simulink model "Linearni"  (R2023b)
settings: Solver=VariableStepAuto  StartTime=0.0  StopTime=stepp.sim_time  RelTol=1e-3
undefined symbols (not defined in the file): ccm_op, dcm_op_cv, G_ccm, Gp_dcm_cv, stepp
settings Model: Creator=teo  LastModifiedBy=teo

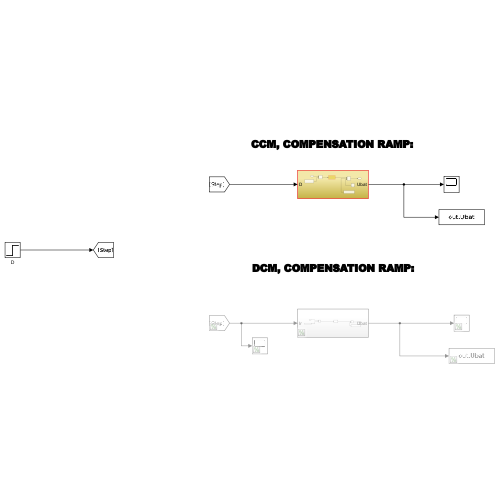
[thumbnail: Simulink's stored preview of the top-level diagram]
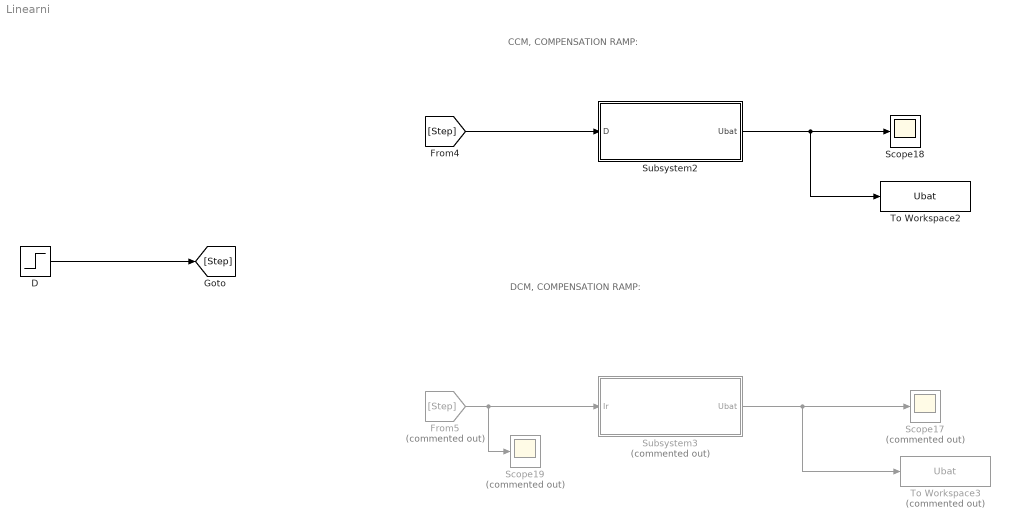
== system Linearni ==
  note: CCM, COMPENSATION RAMP:
  note: DCM, COMPENSATION RAMP:
  D : Step  Time=stepp.step_time  Before=stepp.D1  After=stepp.D2  SampleTime=0
  From5 : From  Commented=on  GotoTag=Step
  Scope17 : Scope  Commented=on
  Scope18 : Scope
  Scope19 : Scope  Commented=on
  Subsystem2 : Subsystem
  Subsystem3 : Subsystem  Commented=on
  To Workspace2 : ToWorkspace  VariableName=Ubat  SaveFormat=Timeseries  SampleTime=1e-6
  To Workspace3 : ToWorkspace  Commented=on  VariableName=Ubat  SaveFormat=Timeseries  SampleTime=1e-6
  wires:
  [Step] -> Subsystem2/1(D)
  Subsystem2/1(Ubat) -> Scope18/1, To Workspace2/1
  From5/1 -> Scope19/1, Subsystem3/1(Ir)
  Subsystem3/1(Ubat) -> To Workspace3/1, Scope17/1
  D/1 -> [Step]

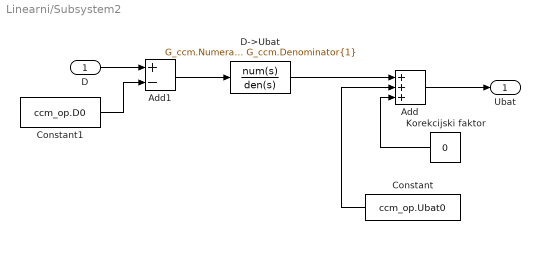
== system Linearni/Subsystem2 ==
  D : Inport
  Add : Sum  Inputs=+++
  Add1 : Sum  Inputs=+-
  Constant : Constant  Value=ccm_op.Ubat0
  Constant1 : Constant  Value=ccm_op.D0
  D->Ubat : TransferFcn  Numerator=G_ccm.Numerator{1}  Denominator=G_ccm.Denominator{1}
  Korekcijski faktor : Constant  Value=0
  Ubat : Outport
  wires:
  D/1 -> Add1/1
  Constant1/1 -> Add1/2
  Add1/1 -> D->Ubat/1
  Add/1 -> Ubat/1
  Constant/1 -> Add/2
  D->Ubat/1 -> Add/1
  Korekcijski faktor/1 -> Add/3

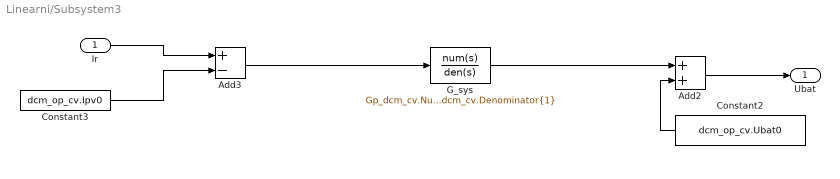
== system Linearni/Subsystem3 ==
  Ir : Inport
  Add2 : Sum
  Add3 : Sum  Inputs=+-
  Constant2 : Constant  Value=dcm_op_cv.Ubat0
  Constant3 : Constant  Value=dcm_op_cv.Ipv0
  G_sys : TransferFcn  Numerator=Gp_dcm_cv.Numerator{1}  Denominator=Gp_dcm_cv.Denominator{1}
  Ubat : Outport
  wires:
  Constant3/1 -> Add3/2
  Add3/1 -> G_sys/1
  G_sys/1 -> Add2/1
  Constant2/1 -> Add2/2
  Ir/1 -> Add3/1
  Add2/1 -> Ubat/1
